simulink model "airspeed_from_pitch_loop"  (Simulink 7.4)
settings: Solver=ode45  StartTime=0.0  StopTime=100  RelTol=1e-3
values from neighbouring files (symbols this model uses):
  a_beta1 = den(2)    [computeGains.m]    (also in compute_tf_model.m = (rho*P.Va*P.S_wing)/2/P.mass*P.C_Y_beta)
  a_beta2 = num(2)    [computeGains.m]    (also in compute_tf_model.m = (rho*P.Va^2*P.S_wing)/2/P.mass*P.C_Y_delta_r)
  delta_r_max = 20*pi/180    (= 0.349065850399)    [computeGains.m]
  P = varargin{5}    [my_mav_dynamics.m]
  vr_max = 3    [computeGains.m]
settings Model: Creator=beard  LastModifiedBy=beard

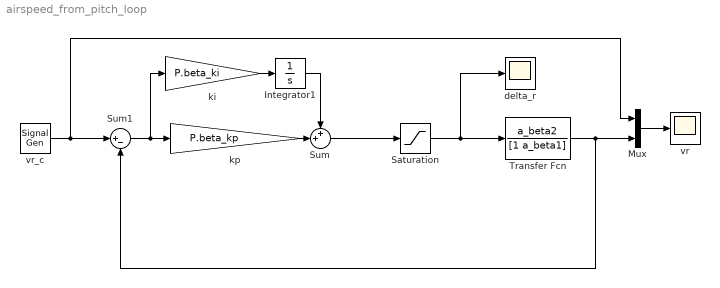
== system airspeed_from_pitch_loop ==
  Integrator1 : Integrator
  Mux : Mux  Inputs=2
  Saturation : Saturate  UpperLimit=delta_r_max  LowerLimit=-delta_r_max  OutDataType=fixdt(1, 16)  OutScaling=2^0
  Sum : Sum  Inputs=++|  OutDataType=fixdt(1, 16)  OutScaling=2^0
  Sum1 : Sum  Inputs=|+-  OutDataType=fixdt(1, 16)  OutScaling=2^0
  Transfer Fcn : TransferFcn  Numerator=a_beta2  Denominator=[1 a_beta1]
  delta_r : Scope
      settings: TimeRange=100  YMin=-3  YMax=3
  ki : Gain  Gain=P.beta_ki  ParameterDataType=fixdt(1, 16)  ParameterScaling=2^0  OutDataType=fixdt(1, 16)  OutScaling=2^0
  kp : Gain  Gain=P.beta_kp  ParameterDataType=fixdt(1, 16)  ParameterScaling=2^0  OutDataType=fixdt(1, 16)  OutScaling=2^0
  vr : Scope
      settings: TimeRange=100  YMin=-3  YMax=3
  vr_c : SignalGenerator  WaveForm=square  Amplitude=vr_max  Frequency=.02
  wires:
  Sum/1 -> Saturation/1
  kp/1 -> Sum/2
  Sum1/1 -> kp/1, ki/1
  ki/1 -> Integrator1/1
  Integrator1/1 -> Sum/1
  vr_c/1 -> Sum1/1, Mux/1
  Mux/1 -> vr/1
  Transfer Fcn/1 -> Sum1/2, Mux/2
  Saturation/1 -> Transfer Fcn/1, delta_r/1
